simulink model "project3"  (R2017a)
settings: Solver=ode3  StartTime=0.0  StopTime=inf  FixedStep=0.001  RelTol=1e-3  EnableMultiTasking=on
libraries: slrtlib x4, xpcquanserlib x2
settings Model: SimulationMode=external  Creator=Ninad  LastModifiedBy=drewkize
settings SolverCC: EnableConcurrentExecution=on
settings DataIOCC: LimitDataPoints=on  SaveFormat=Array  SignalLoggingSaveFormat=ModelDataLogs
settings OptimizationCC: BlockReduction=off  OptimizeBlockIOStorage=off  BufferReuse=off  GlobalBufferReuse=off  ExpressionFolding=off  ExpressionDepthLimit=2147483647  LocalBlockOutputs=off  LifeSpan=inf
settings DebuggingCC: UnderspecifiedInitializationDetection=Classic  MergeDetectMultiDrivingBlocksExec=none  SolverPrmCheckMsg=warning  FcnCallInpInsideContextMsg=warning  StateNameClashWarn=warning  SFUnexpectedBacktrackingDiag=warning  SFNoUnconditionalDefaultTransitionDiag=warning  SFExecutionAtInitializationDiag=none
settings HardwareCC: ProdBitPerPointer=32  ProdBitPerSizeT=32  ProdBitPerPtrDiffT=32  ProdLargestAtomicFloat=None  ProdWordSize=32  ProdLongLongMode=on  ProdHWDeviceType=Generic->32-bit x86 compatible
settings ModelReferenceCC: PropagateSignalLabelsOutOfModel=off
settings RTWCC: SystemTargetFile=slrt.tlc  TemplateMakefile=slrt_default_tmf  Description=Simulink Real-Time  RTWCompilerOptimization=on
settings SimulinkRealTimeCC: GeneratePreprocessorConditionals=Disable all
settings ConfigComp: CovMetricSettings=dw  CovHtmlReporting=on  CovSaveCumulativeToWorkspaceVar=on  CovSaveSingleToWorkspaceVar=on  CovExternalEMLEnable=off  CovSFcnEnable=off

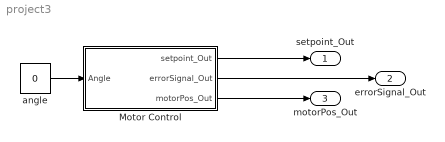
== system project3 ==
  Motor Control : Subsystem
  angle : Constant  Value=0
  setpoint_Out : Outport
  errorSignal_Out : Outport  Port=2
  motorPos_Out : Outport  Port=3
  wires:
  Motor Control/1(setpoint_Out) -> setpoint_Out/1
  Motor Control/2(errorSignal_Out) -> errorSignal_Out/1
  Motor Control/3(motorPos_Out) -> motorPos_Out/1
  angle/1 -> Motor Control/1(Angle)

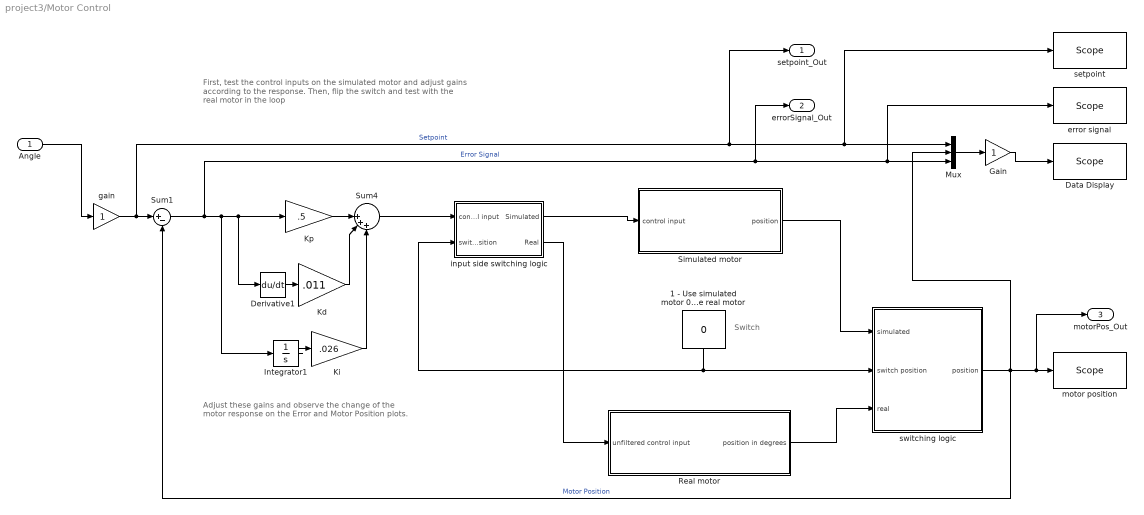
== system project3/Motor Control ==
  note: Adjust these gains and observe the change of the
      | motor response on the Error and Motor Position
      | plots.
  note: First, test the control inputs on the simulated motor and
      | adjust gains according to the response. Then, flip the switch and
      | test with the real motor in the loop
  note: Switch
  Angle : Inport
  1 - Use simulated motor 0 - Use real motor : Constant  Value=0
  Data Display : slrtlib/Displays and Logging/Scope   scopeno=3  scopetype=Target  autostart=on  viewmode=Numerical  formatstr="'Setpoint        %3.2f,Motor Position  %3.2f,Error Signal    %3.2f'"  grid=on  ylimits=[0,170]  nosamples=200  noprepostsamples=0  interleave=10  triggermode=FreeRun  triggersignal=1  trigsignalfromport=off  triggerlevel=0.0  triggerslope=Either  triggerscope=1  triggersample=0  filename=data.dat  mode=Lazy  writesize=512  autorestart=off  dynamicfilemode=off  maxwritefilesize=512*1024^2
  Derivative1 : Derivative
  Gain : Gain
  Integrator1 : Integrator
  Kd : Gain  Gain=.011
  Ki : Gain  Gain=.026
  Kp : Gain  Gain=.5
  Mux : Mux  Inputs=3
  Real motor : Subsystem
  Simulated motor : Subsystem
  Sum1 : Sum  Inputs=|+-
  Sum4 : Sum  Inputs=||+++
  error signal : slrtlib/Displays and Logging/Scope   scopeno=2  scopetype=Target  autostart=on  viewmode=Graphical rolling  formatstr='%15.6f'  grid=on  ylimits=[-180,180]  nosamples=500  noprepostsamples=0  interleave=10  triggermode=FreeRun  triggersignal=1  trigsignalfromport=off  triggerlevel=0.0  triggerslope=Either  triggerscope=1  triggersample=0  filename=data.dat  mode=Lazy  writesize=512  autorestart=off  dynamicfilemode=off  maxwritefilesize=512*1024^2
  gain : Gain
  input side switching logic : Subsystem
  motor position : slrtlib/Displays and Logging/Scope   scopeno=7  scopetype=Target  autostart=on  viewmode=Graphical rolling  formatstr='%15.6f'  grid=on  ylimits=[-180,180]  nosamples=500  noprepostsamples=0  interleave=10  triggermode=FreeRun  triggersignal=1  trigsignalfromport=off  triggerlevel=0.0  triggerslope=Either  triggerscope=1  triggersample=0  filename=data.dat  mode=Lazy  writesize=512  autorestart=off  dynamicfilemode=off  maxwritefilesize=512*1024^2
  setpoint : slrtlib/Displays and Logging/Scope   scopeno=1  scopetype=Target  autostart=on  viewmode=Graphical rolling  formatstr='%15.6f'  grid=on  ylimits=[-180,180]  nosamples=500  noprepostsamples=0  interleave=10  triggermode=FreeRun  triggersignal=1  trigsignalfromport=off  triggerlevel=0.0  triggerslope=Either  triggerscope=1  triggersample=0  filename=data.dat  mode=Lazy  writesize=512  autorestart=off  dynamicfilemode=off  maxwritefilesize=512*1024^2
  switching logic : Subsystem
  setpoint_Out : Outport
  errorSignal_Out : Outport  Port=2
  motorPos_Out : Outport  Port=3
  wires:
  Kp/1 -> Sum4/1
  Kd/1 -> Sum4/2
  Derivative1/1 -> Kd/1
  input side switching logic/1(Simulated) -> Simulated motor/1(control input)
  Mux/1 -> Gain/1
  gain/1 -> Sum1/1, setpoint_Out/1, Mux/1, setpoint/1  "Setpoint"
  Sum4/1 -> input side switching logic/1(control input)
  Real motor/1(position in degrees) -> switching logic/3(real)
  Ki/1 -> Sum4/3
  Simulated motor/1(position) -> switching logic/1(simulated)
  switching logic/1(position) -> Mux/2, Sum1/2, motorPos_Out/1, motor position/1  "Motor Position"
  1 - Use simulated motor 0 - Use real motor/1 -> input side switching logic/2(switch position), switching logic/2(switch position)
  Integrator1/1 -> Ki/1
  Gain/1 -> Data Display/1
  input side switching logic/2(Real) -> Real motor/1(unfiltered control input)
  Sum1/1 -> Kp/1, Derivative1/1, Integrator1/1, errorSignal_Out/1, Mux/3, error signal/1  "Error Signal"
  Angle/1 -> gain/1

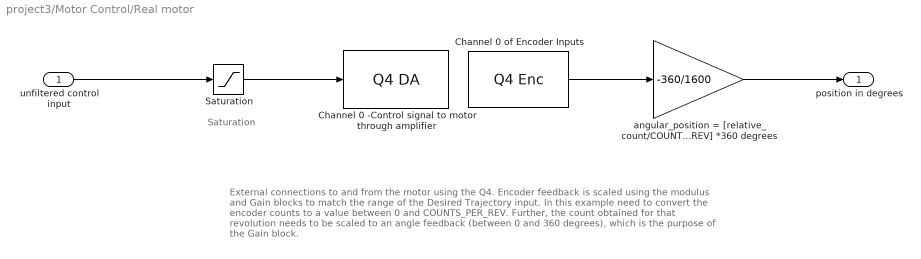
== system project3/Motor Control/Real motor ==
  note: Saturation
  note: External connections to and from the motor using the Q4.
      |
      | Encoder feedback is scaled using the modulus and Gain blocks to
      | match the range of the Desired Trajectory input.
      |
      | In this example need to convert the encoder counts to a value between 0 and COUNTS_PER_REV.
      | Further, the count obtained for that revolution needs to be scaled to an angle feedback (between
      | 0 and 360 degrees), which is the purpose of the Gain block.
  unfiltered control input : Inport
  "Channel 0 -Control signal to motor through amplifier " : xpcquanserlib/D//A/Q4 DA   channel=[1]  range=[-10]  simul=off  reset=[1]  initValue=[0]  sampleTime=.001  slot=-1
      settings: SourceProductName=Simulink Real-Time  SourceProductBaseCode=XP
  "Channel 0 of Encoder Inputs " : xpcquanserlib/Incremental Encoder/Q4 Enc   channel=[1]  initialCount=[0]  prescale=[1]  quadrature=[4]  mode=[0]  synchronousIndex=[0]  indexPolarity=[0]  preserveCounts=[0]  sampleTime=.001  slot=-1
      settings: SourceProductName=Simulink Real-Time  SourceProductBaseCode=XP
  Saturation : Saturate  UpperLimit=10  LowerLimit=-10
  angular_position = [relative_count/COUNTS_PER_REV] *360 degrees : Gain  Gain=-360/1600
  position in degrees : Outport
  wires:
  Saturation/1 -> "Channel 0 -Control signal to motor through amplifier "/1
  angular_position = [relative_count/COUNTS_PER_REV] *360 degrees/1 -> position in degrees/1
  "Channel 0 of Encoder Inputs "/1 -> angular_position = [relative_count/COUNTS_PER_REV] *360 degrees/1
  unfiltered control input/1 -> Saturation/1

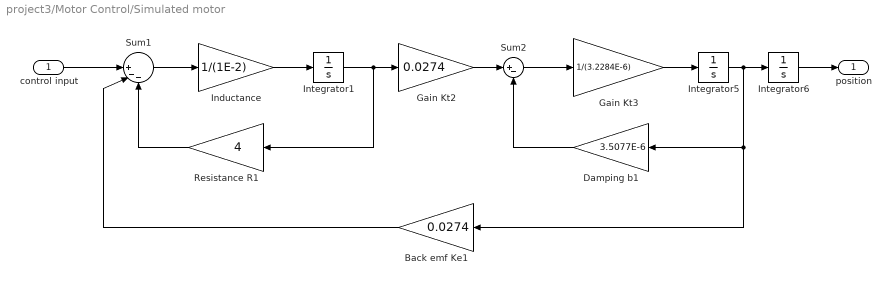
== system project3/Motor Control/Simulated motor ==
  control input : Inport
  Back emf Ke1 : Gain  Gain=0.0274
  Damping b1 : Gain  Gain=3.5077E-6
  Gain Kt2 : Gain  Gain=0.0274
  Gain Kt3 : Gain  Gain=1/(3.2284E-6)
  Inductance : Gain  Gain=1/(1E-2)
  Integrator1 : Integrator
  Integrator5 : Integrator
  Integrator6 : Integrator
  Resistance R1 : Gain  Gain=4
  Sum1 : Sum  Inputs=||+--
  Sum2 : Sum  Inputs=|+-
  position : Outport
  wires:
  Sum1/1 -> Inductance/1
  Inductance/1 -> Integrator1/1
  Integrator1/1 -> Gain Kt2/1, Resistance R1/1
  Gain Kt2/1 -> Sum2/1
  Sum2/1 -> Gain Kt3/1
  Gain Kt3/1 -> Integrator5/1
  Integrator5/1 -> Integrator6/1, Back emf Ke1/1, Damping b1/1
  Back emf Ke1/1 -> Sum1/2
  Damping b1/1 -> Sum2/2
  Resistance R1/1 -> Sum1/3
  Integrator6/1 -> position/1
  control input/1 -> Sum1/1

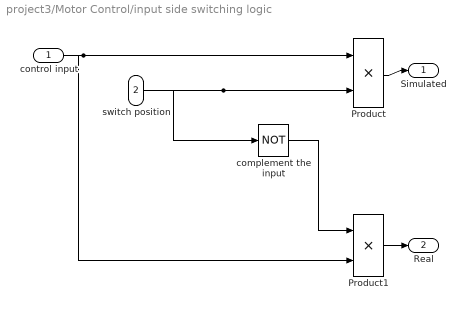
== system project3/Motor Control/input side switching logic ==
  control input : Inport
  switch position : Inport  Port=2
  Product : Product  RndMeth=Zero
  Product1 : Product  RndMeth=Zero
  complement the input : Logic  Operator=NOT  AllPortsSameDT=off  OutDataTypeStr=boolean
  Simulated : Outport
  Real : Outport  Port=2
  wires:
  control input/1 -> Product1/2, Product/1
  complement the input/1 -> Product1/1
  switch position/1 -> complement the input/1, Product/2
  Product/1 -> Simulated/1
  Product1/1 -> Real/1

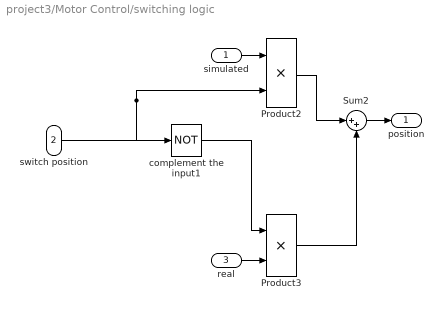
== system project3/Motor Control/switching logic ==
  simulated : Inport
  switch position : Inport  Port=2
  real : Inport  Port=3
  Product2 : Product  RndMeth=Zero
  Product3 : Product  RndMeth=Zero
  Sum2 : Sum  Inputs=|++
  complement the input1 : Logic  Operator=NOT  AllPortsSameDT=off  OutDataTypeStr=boolean
  position : Outport
  wires:
  complement the input1/1 -> Product3/1
  Product2/1 -> Sum2/1
  Product3/1 -> Sum2/2
  switch position/1 -> complement the input1/1, Product2/2
  simulated/1 -> Product2/1
  Sum2/1 -> position/1
  real/1 -> Product3/2
